simulink subsystem "Sub_VehicleModel"  (R2021b)
settings: Solver=VariableStepAuto  StartTime=0.0  StopTime=10.0  RelTol=1e-3
undefined symbols (not defined in the file): Ts, v0_ego, x0_ego
libraries: commrandsrc3 x1
settings Model: Creator=Otonom  LastModifiedBy=Otonom

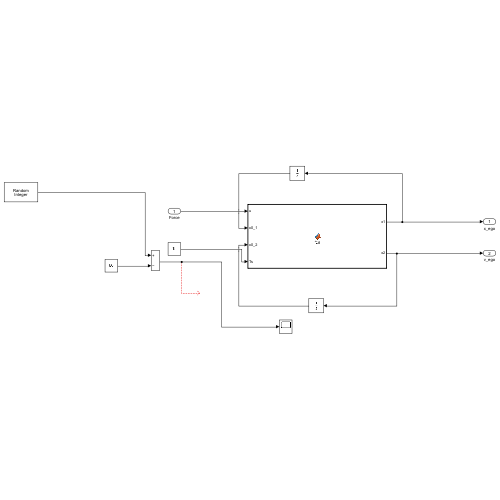
[thumbnail: Simulink's stored preview of the top-level diagram]
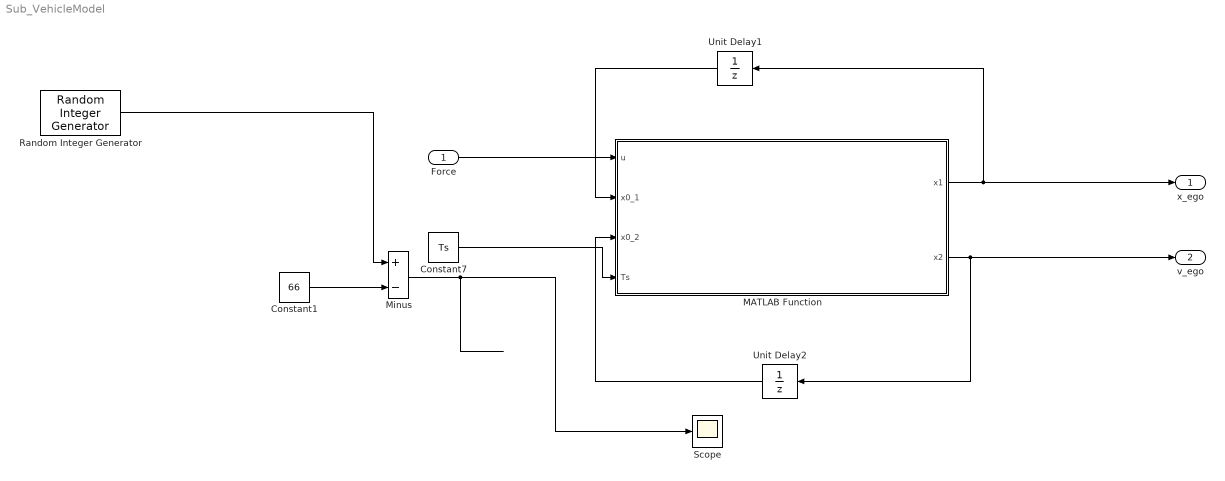
== system Sub_VehicleModel ==
  Force : Inport
  Constant1 : Constant  Value=66
  Constant7 : Constant  Value=Ts
  MATLAB Function : MATLAB Function  TreatAsAtomicUnit=on
  Minus : Sum  Inputs=+-
  Random Integer Generator : commrandsrc3/Random Integer Generator  SetSize=150  SeedSource=Auto  Seed=0  SampleTime=0.1  SamplesPerFrame=1  OutputDataType=double  SimulateUsing=Interpreted execution
  Scope : Scope
  Unit Delay1 : UnitDelay  InitialCondition=x0_ego  SampleTime=-1  HasFrameUpgradeWarning=on
  Unit Delay2 : UnitDelay  InitialCondition=v0_ego  SampleTime=-1  HasFrameUpgradeWarning=on
  x_ego : Outport
  v_ego : Outport  Port=2
  wires:
  Random Integer Generator/1 -> Minus/1
  Constant1/1 -> Minus/2
  Minus/1 -> Scope/1
  MATLAB Function/1(x1) -> x_ego/1, Unit Delay1/1
  Unit Delay1/1 -> MATLAB Function/2(x0_1)
  Unit Delay2/1 -> MATLAB Function/3(x0_2)
  Force/1 -> MATLAB Function/1(u)
  MATLAB Function/2(x2) -> v_ego/1, Unit Delay2/1
  Constant7/1 -> MATLAB Function/4(Ts)

== matlab function Sub_VehicleModel/MATLAB Function ==
  data: u input; x1 output; x0_1 input; x0_2 input; x2 output; Ts input
function [x1, x2] = fcn(u, x0_1, x0_2, Ts)
    m = 4700;
    b = 444;
    delta = Ts;

    A_init = [0 1.0000; 0 -b/m];
    B_init = [0; 1/m];

    A = A_init * delta + eye(2);
    B = B_init * delta;
    C = [1 0];

    x0 = [x0_1; x0_2];
    y = A * x0 + B * u;

    x1 = y(1);
    x2 = y(2);
end
